simulink model "node_model"  (R2020a)
settings: Solver=FixedStepAuto  StartTime=0.0  StopTime=50  FixedStep=1e-3  RelTol=1e-3
undefined symbols (not defined in the file): Initial_Voltages, Max_energy_threshold, Min_energy_threshold, NUM_NODES
settings Model: Creator=赵一泽  LastModifiedBy=赵一泽
settings DataIOCC: ReturnWorkspaceOutputs=off
settings DebuggingCC: UnconnectedInputMsg=none  UnconnectedOutputMsg=none  UnconnectedLineMsg=none
settings ModelReferenceCC: EnableRefExpFcnMdlSchedulingChecks=off
settings RTWCC: Description=Generic Real-Time Target

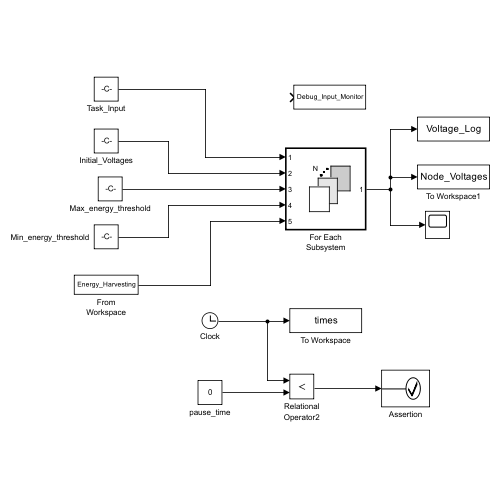
[thumbnail: Simulink's stored preview of the top-level diagram]
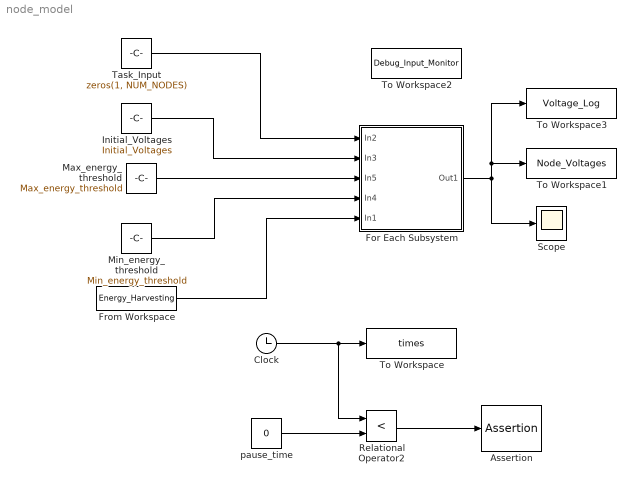
== system node_model ==
  Assertion : Assertion  AssertionFailFcn=set_param(bdroot, 'simulationCommand', 'pause')  StopWhenAssertionFail=off
  Clock : Clock
  For Each Subsystem : Subsystem  TreatAsAtomicUnit=on
  From Workspace : FromWorkspace  VariableName=Energy_Harvesting
  Initial_Voltages : Constant  Value=Initial_Voltages
  Max_energy_threshold : Constant  Value=Max_energy_threshold
  Min_energy_threshold : Constant  Value=Min_energy_threshold
  Relational Operator2 : RelationalOperator  Operator=<  OutDataTypeStr=boolean  RndMeth=Simplest
  Scope : Scope
  Task_Input : Constant  Value=zeros(1, NUM_NODES)
  To Workspace : ToWorkspace  VariableName=times  SampleTime=-1
  To Workspace1 : ToWorkspace  VariableName=Node_Voltages  SampleTime=-1
      settings: MaxDataPoints=1
  To Workspace2 : ToWorkspace  VariableName=Debug_Input_Monitor  SampleTime=-1
      settings: MaxDataPoints=1
  To Workspace3 : ToWorkspace  VariableName=Voltage_Log  SaveFormat=Structure With Time  SampleTime=-1
  pause_time : Constant  Value=0
  wires:
  pause_time/1 -> Relational Operator2/2
  Relational Operator2/1 -> Assertion/1
  Clock/1 -> Relational Operator2/1, To Workspace/1
  Task_Input/1 -> For Each Subsystem/1(In2)
  Initial_Voltages/1 -> For Each Subsystem/2(In3)
  For Each Subsystem/1(Out1) -> To Workspace3/1, To Workspace1/1, Scope/1
  From Workspace/1 -> For Each Subsystem/5(In1)
  Min_energy_threshold/1 -> For Each Subsystem/4(In4)
  Max_energy_threshold/1 -> For Each Subsystem/3(In5)

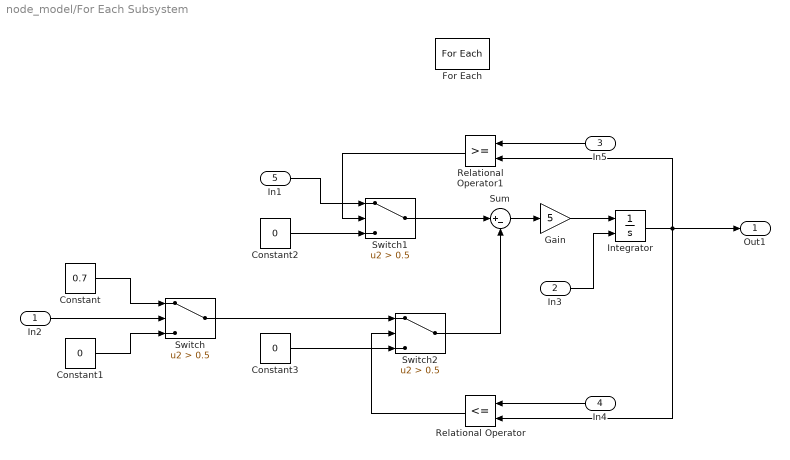
== system node_model/For Each Subsystem ==
  In2 : Inport  Partition=on  PartitionDimension=1  PartitionWidth=NUM_NODES  PartitionOffset=0
  In3 : Inport  Port=2  Partition=on  PartitionDimension=1  PartitionWidth=NUM_NODES  PartitionOffset=0
  In5 : Inport  Port=3
  In4 : Inport  Port=4
  In1 : Inport  Port=5  Partition=on  PartitionDimension=1  PartitionWidth=NUM_NODES  PartitionOffset=0
  Constant : Constant  Value=0.7
  Constant1 : Constant  Value=0
  Constant2 : Constant  Value=0
  Constant3 : Constant  Value=0
  For Each : ForEach  DisableCoverage=on
  Gain : Gain  Gain=5
  Integrator : Integrator  InitialConditionSource=external  LimitOutput=on  UpperSaturationLimit=4.3  LowerSaturationLimit=0
  Relational Operator : RelationalOperator  Operator=<=  OutDataTypeStr=boolean  RndMeth=Simplest
  Relational Operator1 : RelationalOperator  OutDataTypeStr=boolean  RndMeth=Simplest
  Sum : Sum  Inputs=|+-
  Switch : Switch  Criteria=u2 > Threshold  Threshold=0.5
  Switch1 : Switch  Criteria=u2 > Threshold  Threshold=0.5
  Switch2 : Switch  Criteria=u2 > Threshold  Threshold=0.5
  Out1 : Outport  ConcatenationDimension=1
  wires:
  In2/1 -> Switch/2
  Constant/1 -> Switch/1
  Constant1/1 -> Switch/3
  Sum/1 -> Gain/1
  Gain/1 -> Integrator/1
  In3/1 -> Integrator/2
  Integrator/1 -> Relational Operator1/2, Relational Operator/2, Out1/1
  Constant2/1 -> Switch1/3
  Switch1/1 -> Sum/1
  In1/1 -> Switch1/1
  In5/1 -> Relational Operator1/1
  Relational Operator1/1 -> Switch1/2
  Switch2/1 -> Sum/2
  Relational Operator/1 -> Switch2/2
  In4/1 -> Relational Operator/1
  Constant3/1 -> Switch2/3
  Switch/1 -> Switch2/1
